simulink model "BatteryTestHarness"  (R2024b)
settings: Solver=VariableStepAuto  StartTime=0.0  StopTime=1200  RelTol=1e-3
libraries: fl_lib x9, nesl_utility x5, simulink x3
settings Model: Creator=jjha  LastModifiedBy=jjha
settings OptimizationCC: ReuseModelBlockBuffer=off
settings RTWCC: GPUComputeCapability=3.5

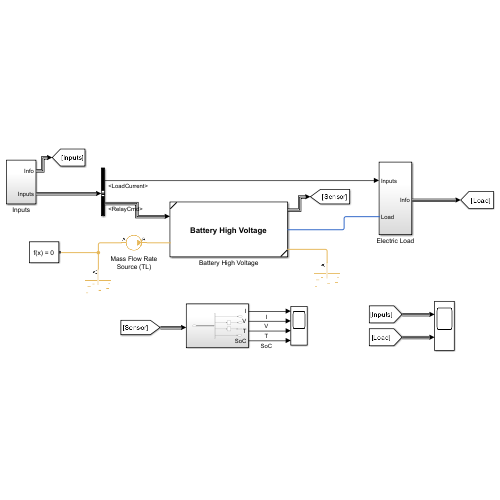
[thumbnail: Simulink's stored preview of the top-level diagram]
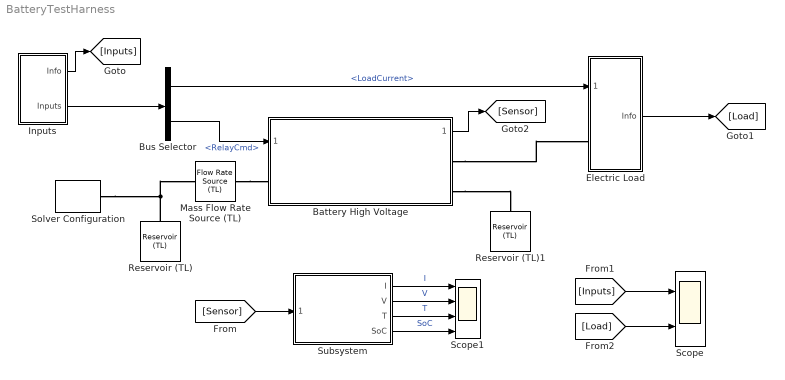
== system BatteryTestHarness ==
  Battery High Voltage : Subsystem  ReferencedSubsystem=BatteryLumpedThermal
      settings: PortSchema="{\"entries\":[{\"content\":{\"sides\":[{\"content\":{\"connectorIds\":[\"In1\",\"LConn1\"]},\"type\":\"ConnectorPlacement.EquallySpacedRectSide\",\"uuid\":\"8181cb02-9fda-4117-b6cc-20d3aa3c91ff\"},{\"content\":{\"connectorIds\":[\"Out1\",\"RConn2\",\"RConn1\"],\"side\":\"RIGHT\"},\"type\":\"ConnectorPlacement.EquallySpacedRectSide\",\"uuid\":\"ce8e42be-3e70-4380-b57d-83f3b727ba87\"},{\"content\":{\"side\":\"TOP\"},\"type\":\"ConnectorPlacement.EquallySpacedRectSide\",\"uuid\":\"6a78c74e-aae9-47cc-a28b-5eba05e58917\"}]},\"type\":\"ConnectorPlacement.EquallySpacedConnector\",\"uuid\":\"1e62e78b-c719-4766-a217-65142f12f1bd\"}],\"packageUris\":[\"http://schema.mathworks.com/mf0/Connector/R2020b\"],\"version\":\"1.0\"}"
  Bus Selector : BusSelector  OutputSignals=Load.LoadCurrent,RelayCmd
  Electric Load : Subsystem
  Inputs : Subsystem
  Mass Flow Rate Source (TL) : fl_lib/Thermal Liquid/Sources/Flow Rate Source (TL)  source_type=foundation.enum.constant_controlled.constant  flow_type=foundation.enum.mass_volumetric_flow.mass  mass_flow=0.001 kg/s  volumetric_flow=0 m^3/s  power_spec=foundation.enum.power_spec.isentropic  area=0.01 m^2
      settings: InternalSimscapePortConfiguration="{\"Bottom\":[],\"Left\":[{\"id\":\"A\",\"label\":\"A\",\"type\":\"foundation.thermal_liquid.thermal_liquid\"}],\"Right\":[{\"id\":\"B\",\"label\":\"B\",\"type\":\"foundation.thermal_liquid.thermal_liquid\"}],\"Top\":[]}"
  Reservoir (TL) : fl_lib/Thermal Liquid/Elements/Reservoir (TL)  pressure_spec=foundation.enum.pressure_spec.atmospheric  reservoir_pressure=0.101325 MPa  reservoir_temperature=293.15 K  area=0.01 m^2
  Reservoir (TL)1 : fl_lib/Thermal Liquid/Elements/Reservoir (TL)  pressure_spec=foundation.enum.pressure_spec.atmospheric  reservoir_pressure=0.101325 MPa  reservoir_temperature=293.15 K  area=0.01 m^2
  Scope : Scope  NumInputPorts=2
  Scope1 : Scope  NumInputPorts=4
  Solver Configuration : nesl_utility/Solver Configuration  PhysicalDomain=network_engine_domain  SubClassName=solver  LeftPortType=input  RightPortType=generic  Tones=[]  Harmonics=[]  SimulateNoise=off  Profile=off  UseLocalSampling=off  EnableSwitchedLinearOptims=on  FrequencyDomain=off  UseCCode=off  RelTol=0.001  AbsTol=0.001  MinStep=1e-09  ToWorkspace=off  RevertToSquareIcSolve=off  NumHomotopyIterations=100  PhasorMode=off  PhasorModeNumHarmonics=1  ConsistencySolver=NEWTON_XTOL_AFTER_FTOL  IndexReductionMethod=DerivativeReplacement  DoDC=off  ResidualTolerance=1e-09  ConsistencyTolSource=GLOBAL  ConsistencyAbsTol=0.001  ConsistencyRelTol=0.001  ConsistencyTolFactor=0.001  UseLocalSolver=off  LocalSolverChoice=NE_BACKWARD_EULER_ADVANCER  ResolveIndetEquations=on  FunctionEvalNumThread=1  LocalSolverSampleTime=0.001  DoFixedCost=off  MaxNonlinIter=3  MaxModeIter=2  ComputeImpulses=off  ImpulseIterations=2  LinearAlgebra=auto  LinearAlgebraNumThread=0  EquationFormulation=NE_TIME_EF  DelaysMemoryBudget=1024  AutomaticFiltering=on  FilteringTimeConstant=0.001  PartitionStorageMethod=AS_NEEDED  PartitionMemoryBudget=1024  PartitionMethod=ROBUST  MultibodyUseLocalSolver=off  MultibodyLocalSolverChoice=ODE1  MultibodyLocalSolverSampleTime=0.001
  Subsystem : Subsystem
  wires:
  Inputs/2(Inputs) -> Bus Selector/1
  Bus Selector/2 -> Battery High Voltage/1  "<RelayCmd>"
  Bus Selector/1 -> Electric Load/1(Inputs)  "<LoadCurrent>"
  Inputs/1(Info) -> [Inputs]
  Electric Load/1(Info) -> [Load]
  Battery High Voltage/1 -> [Sensor]
  [Inputs] -> Scope/1
  [Load] -> Scope/2
  [Sensor] -> Subsystem/1(" ")
  Subsystem/1(I) -> Scope1/1  "I"
  Subsystem/2(V) -> Scope1/2  "V"
  Subsystem/3(T) -> Scope1/3  "T"
  Subsystem/4(SoC) -> Scope1/4  "SoC"
  connections:
  Battery High Voltage/RConn2 -- Electric Load/LConn1
  Mass Flow Rate Source (TL)/RConn1 -- Battery High Voltage/LConn1
  Battery High Voltage/RConn1 -- Reservoir (TL)1/LConn1
  Reservoir (TL)/LConn1 -- Solver Configuration/RConn1 -- Mass Flow Rate Source (TL)/LConn1

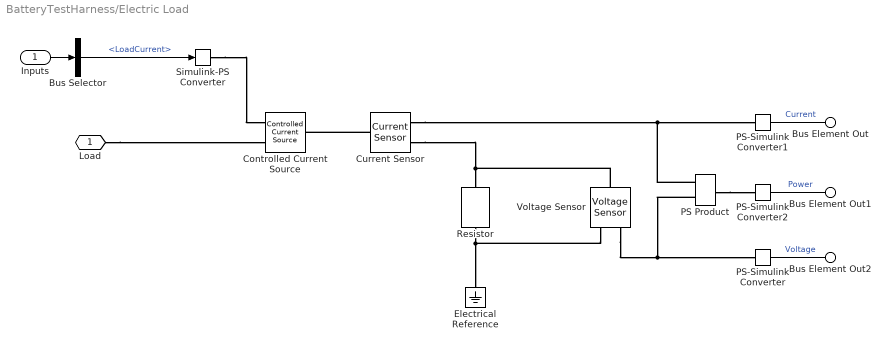
== system BatteryTestHarness/Electric Load ==
  Inputs : Inport
  Bus Selector : BusSelector  OutputSignals=LoadCurrent
  Controlled Current Source : fl_lib/Electrical/Electrical Sources/Controlled Current Source
  Current Sensor : fl_lib/Electrical/Electrical Sensors/Current Sensor
  Electrical Reference : fl_lib/Electrical/Electrical Elements/Electrical Reference
  PS Product : fl_lib/Physical Signals/Functions/PS Product
  PS-Simulink Converter : nesl_utility/PS-Simulink Converter  PhysicalDomain=network_engine_domain  SubClassName=ps_output  LeftPortType=input  RightPortType=output  PseudoPeriodic=off  Frequencies=[]  VectorFormat=inherit  Unit=V  AffineConversion=off
  PS-Simulink Converter1 : nesl_utility/PS-Simulink Converter  PhysicalDomain=network_engine_domain  SubClassName=ps_output  LeftPortType=input  RightPortType=output  PseudoPeriodic=off  Frequencies=[]  VectorFormat=inherit  Unit=A  AffineConversion=off
  PS-Simulink Converter2 : nesl_utility/PS-Simulink Converter  PhysicalDomain=network_engine_domain  SubClassName=ps_output  LeftPortType=input  RightPortType=output  PseudoPeriodic=off  Frequencies=[]  VectorFormat=inherit  Unit=kW  AffineConversion=off
  Resistor : fl_lib/Electrical/Electrical Elements/Resistor  R=1 Ohm  i_specify=off  i_priority=None  i=0 A  i_nominal_specify=off  i_nominal_value=1  i_nominal_unit=A  v_specify=off  v_priority=None  v=0 V  v_nominal_specify=off  v_nominal_value=1  v_nominal_unit=V
  Simulink-PS Converter : nesl_utility/Simulink-PS Converter  PhysicalDomain=network_engine_domain  SubClassName=ps_input  LeftPortType=input  RightPortType=output  PseudoPeriodic=off  Frequencies=[]  NoiseDistribution=none  NoiseParameters=[]  Unit=A  AffineConversion=off  FilteringAndDerivatives=provide  SimscapeFilterOrder=1  InputFilterTimeConstant=0.001  UdotUserProvided=0
  Voltage Sensor : fl_lib/Electrical/Electrical Sensors/Voltage Sensor
  Load : PMIOPort  Side=Left
  Bus Element Out : Outport  PortName=Info  Element=Curr
  Bus Element Out1 : Outport  PortName=Info  Element=Pwr
  Bus Element Out2 : Outport  PortName=Info  Element=V
  wires:
  PS-Simulink Converter1/1 -> Bus Element Out/1  "Current"
  PS-Simulink Converter2/1 -> Bus Element Out1/1  "Power"
  PS-Simulink Converter/1 -> Bus Element Out2/1  "Voltage"
  Inputs/1 -> Bus Selector/1
  Bus Selector/1 -> Simulink-PS Converter/1  "<LoadCurrent>"
  connections:
  Load/RConn1 -- Controlled Current Source/RConn2
  Resistor/RConn1 -- Electrical Reference/LConn1 -- Voltage Sensor/RConn2
  Simulink-PS Converter/RConn1 -- Controlled Current Source/RConn1
  Current Sensor/LConn1 -- Controlled Current Source/LConn1
  Current Sensor/RConn2 -- Voltage Sensor/LConn1 -- Resistor/LConn1
  Voltage Sensor/RConn1 -- PS Product/LConn2 -- PS-Simulink Converter/LConn1
  Current Sensor/RConn1 -- PS Product/LConn1 -- PS-Simulink Converter1/LConn1
  PS Product/RConn1 -- PS-Simulink Converter2/LConn1

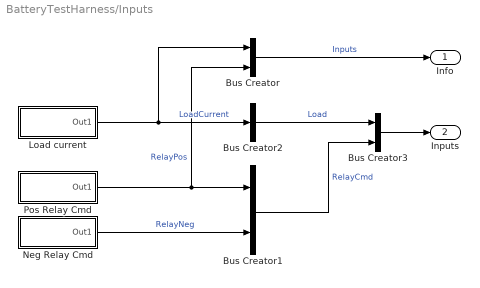
== system BatteryTestHarness/Inputs ==
  Bus Creator : BusCreator  Inputs=2
  Bus Creator1 : BusCreator  Inputs=2
  Bus Creator2 : BusCreator  Inputs=1
  Bus Creator3 : BusCreator  Inputs=2
  Load current : Subsystem  mask(Continuous Multi-Step Signal){dataPoints=[0 5 0;16 114 5;137 256 5;268 378 2;402 479 14;496 579 5;593 660 28;675 787 4;809 901 17;919 1037 25;1049 1137 26;1147 1157 0], deltaT=0.5}
      mask prompts: dataPoints "Data points"; deltaT "Interpolation step [s]"
      mask help:
      | This block generates a signal consisting of smoothly connected flat segments. Data points parameter takes an N-by-3 matrix where each row specifies a flat segment. First column and second column define start and end time of the segment, respectively. Third column defines the value of the segment. Second column can also be NaN to define a point value. Flat segments and point values are smoothly interpolated by Akima spline with the specified interpolation step.
      |
      | For example, a matrix [0 1 5; 3 nan 9; 6 8 7] for Data points defines a signal as follows. First row defines a flat segment from t=0 to t=1 of value 5. Second row defines a point at t=3 of value 9. Third row defines a flat segment from t=6 to t=8 of value 7.
      mask init:
      | sig = SignalDesigner("ContinuousMultiStep");
      | 
      | % Initialization function can access parameter names directly
      | sig.XYData = dataPoints;
      | sig.DeltaX = deltaT;
      | 
      | update(sig)
      | 
      | SignalSourceBlockCallback.setDataToLookupTableBlock( ...
      |   SignalObject = sig, ...
      |   PathToBlock = [gcb '/1-D Lookup Table']);
      mask DialogControl Control3 Prompt: horizontal spacer 1
      mask DialogControl Control4 Prompt: horizontal spacer 2
      mask DialogControl Control5 Prompt: horizontal spacer 3
      mask DialogControl PlotButton Prompt: Plot
      mask DialogControl PlotButton Callback: SignalSourceBlockCallback.plotContinuousMultiStep(gcb);
      mask Display: disp("Continuous" + newline + "Multi-Step")
  Neg Relay Cmd : Subsystem  mask(Continuous Multi-Step Signal){dataPoints=[0 1 0;2 10 1], deltaT=0.1}
      mask prompts: dataPoints "Data points"; deltaT "Interpolation step [s]"
      mask help:
      | This block generates a signal consisting of smoothly connected flat segments. Data points parameter takes an N-by-3 matrix where each row specifies a flat segment. First column and second column define start and end time of the segment, respectively. Third column defines the value of the segment. Second column can also be NaN to define a point value. Flat segments and point values are smoothly interpolated by Akima spline with the specified interpolation step.
      |
      | For example, a matrix [0 1 5; 3 nan 9; 6 8 7] for Data points defines a signal as follows. First row defines a flat segment from t=0 to t=1 of value 5. Second row defines a point at t=3 of value 9. Third row defines a flat segment from t=6 to t=8 of value 7.
      mask init: same as BatteryTestHarness/Inputs/Load current
      mask DialogControl Control3 Prompt: horizontal spacer 1
      mask DialogControl Control4 Prompt: horizontal spacer 2
      mask DialogControl Control5 Prompt: horizontal spacer 3
      mask DialogControl PlotButton Prompt: Plot
      mask DialogControl PlotButton Callback: SignalSourceBlockCallback.plotContinuousMultiStep(gcb);
      mask Display: disp("Continuous" + newline + "Multi-Step")
  Pos Relay Cmd : Subsystem  mask(Continuous Multi-Step Signal){dataPoints=[0 1 0;2 10 1], deltaT=0.1}
      mask prompts: dataPoints "Data points"; deltaT "Interpolation step [s]"
      mask help:
      | This block generates a signal consisting of smoothly connected flat segments. Data points parameter takes an N-by-3 matrix where each row specifies a flat segment. First column and second column define start and end time of the segment, respectively. Third column defines the value of the segment. Second column can also be NaN to define a point value. Flat segments and point values are smoothly interpolated by Akima spline with the specified interpolation step.
      |
      | For example, a matrix [0 1 5; 3 nan 9; 6 8 7] for Data points defines a signal as follows. First row defines a flat segment from t=0 to t=1 of value 5. Second row defines a point at t=3 of value 9. Third row defines a flat segment from t=6 to t=8 of value 7.
      mask init: same as BatteryTestHarness/Inputs/Load current
      mask DialogControl Control3 Prompt: horizontal spacer 1
      mask DialogControl Control4 Prompt: horizontal spacer 2
      mask DialogControl Control5 Prompt: horizontal spacer 3
      mask DialogControl PlotButton Prompt: Plot
      mask DialogControl PlotButton Callback: SignalSourceBlockCallback.plotContinuousMultiStep(gcb);
      mask Display: disp("Continuous" + newline + "Multi-Step")
  Info : Outport
  Inputs : Outport  Port=2
  wires:
  Load current/1(Out1) -> Bus Creator2/1, Bus Creator/1  "LoadCurrent"
  Pos Relay Cmd/1(Out1) -> Bus Creator1/1, Bus Creator/2  "RelayPos"
  Bus Creator/1 -> Info/1  "Inputs"
  Bus Creator2/1 -> Bus Creator3/1  "Load"
  Bus Creator1/1 -> Bus Creator3/2  "RelayCmd"
  Bus Creator3/1 -> Inputs/1
  Neg Relay Cmd/1(Out1) -> Bus Creator1/2  "RelayNeg"

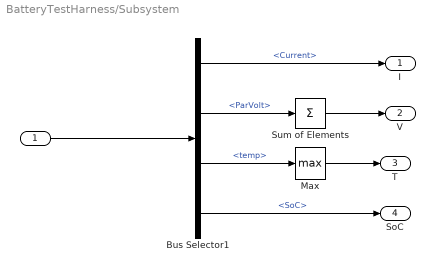
== system BatteryTestHarness/Subsystem ==
  " " : Inport
  Bus Selector1 : BusSelector  OutputSignals=BattSens.Current,BattSens.ParVolt,BattSens.temp,BattSens.SoC
  Max : MinMax  Function=max  ZeroCross=off
  Sum of Elements : Sum  Inputs=+
  I : Outport
  V : Outport  Port=2
  T : Outport  Port=3
  SoC : Outport  Port=4
  wires:
  " "/1 -> Bus Selector1/1
  Bus Selector1/1 -> I/1  "<Current>"
  Bus Selector1/2 -> Sum of Elements/1  "<ParVolt>"
  Bus Selector1/3 -> Max/1  "<temp>"
  Bus Selector1/4 -> SoC/1  "<SoC>"
  Sum of Elements/1 -> V/1
  Max/1 -> T/1

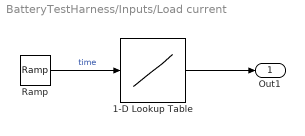
== system BatteryTestHarness/Inputs/Load current ==
  1-D Lookup Table : Lookup_n-D  NumberOfTableDimensions=1  BreakpointsForDimension1="[0              5            5.5              6            6.5              7            7.5              8            8.5              9            9.5             10           10.5             11           11.5             12           12.5             13           13.5             14           14.5             15           15.5             16            114          114.5            115          115.5            116          116.5            117          117.5            118          118.5            119          119.5            120          120.5            121          121.5            122          122.5            123          123.5            124          124.5            125          125.5            126          126.5            127          127.5            128          128.5            129          129.5            130          130.5            131          131.5            132          132.5            133          133.5            134          134.5            135          135.5            136          136.5            137            256          256.5            257          257.5            258          258.5            259          259.5            260          260.5            261          261.5            262          262.5            263          263.5            264          264.5            265          265.5            266          266.5            267          267.5            268            378          378.5            379          379.5            380          380.5            381          381.5            382          382.5            383          383.5            384          384.5            385          385.5            386          386.5            387          387.5            388          388.5            389          389.5            390          390.5            391          391.5            392          392.5            393          393.5            394          394.5            395          395.5            396          396.5            397          397.5            398          398.5            399          399.5            400          400.5            401          401.5            402            479          479.5            480          480.5            481          481.5            482          482.5            483          483.5            484          484.5            485          485.5            486          486.5            487          487.5            488          488.5            489          489.5            490          490.5            491          491.5            492          492.5            493          493.5            494          494.5            495          495.5            496            579          579.5            580          580.5            581          581.5            582          582.5            583          583.5            584          584.5            585          585.5            586          586.5            587          587.5            588          588.5            589          589.5            590          590.5            591          591.5            592          592.5            593            660          660.5            661          661.5            662          662.5            663          663.5            664          664.5            665          665.5            666          666.5            667          667.5            668          668.5            669          669.5            670          670.5            671          671.5            672          672.5            673          673.5            674          674.5            675            787          787.5            788          788.5            789          789.5            790          790.5            791          791.5            792          792.5            793          793.5            794          794.5            795          795.5            796          796.5            797          797.5            798          798.5            799          799.5            800 ...(+1523 chars)]"  Table="[0            0    0.0300526     0.116454     0.253569     0.435763       0.6574     0.912847      1.19647      1.50263      1.82569      2.16003          2.5      2.83997      3.17431      3.49737      3.80353      4.08715       4.3426      4.56424      4.74643      4.88355      4.96995            5            5            5            5            5            5            5            5            5            5            5            5            5            5            5            5            5            5            5            5            5            5            5            5            5            5            5            5            5            5            5            5            5            5            5            5            5            5            5            5            5            5            5            5            5            5            5            5            5      4.98481      4.94097      4.87109      4.77778      4.66363      4.53125      4.38325      4.22222      4.05078      3.87153      3.68707          3.5      3.31293      3.12847      2.94922      2.77778      2.61675      2.46875      2.33637      2.22222      2.12891      2.05903      2.01519            2            2      2.01541      2.06076      2.13477      2.23611       2.3635      2.51562      2.69119      2.88889      3.10742      3.34549      3.60178        3.875      4.16385      4.46701       4.7832      5.11111      5.44944      5.79688      6.15213      6.51389      6.88086      7.25174      7.62522            8      8.37478      8.74826      9.11914      9.48611      9.84787      10.2031      10.5506      10.8889      11.2168       11.533      11.8362       12.125      12.3982      12.6545      12.8926      13.1111      13.3088      13.4844      13.6365      13.7639      13.8652      13.9392      13.9846           14           14      13.9771      13.9102      13.8022      13.6556      13.4733      13.2581      13.0126      12.7397       12.442      12.1223      11.7834       11.428      11.0589      10.6788      10.2905       9.8966          9.5       9.1034      8.70955      8.32119      7.94107      7.57195      7.21657      6.87767      6.55801      6.26033      5.98738      5.74191      5.52666      5.34439      5.19784      5.08976       5.0229            5            5      5.08591      5.33528      5.73551      6.27405      6.93832      7.71574      8.59375      9.55977      10.6012      11.7055      12.8601      14.0525        15.27         16.5        17.73      18.9475      20.1399      21.2945      22.3988      23.4402      24.4062      25.2843      26.0617      26.7259      27.2645      27.6647      27.9141           28           28      27.9218      27.6942       27.328      26.8338      26.2222       25.504      24.6898      23.7902       22.816      21.7778      20.6862       19.552      18.3858      17.1982           16      14.8018      13.6142       12.448      11.3138      10.2222        9.184      8.20978      7.31022        6.496      5.77778      5.16622        4.672      4.30578      4.07822            4            4      4.01984      4.07814      4.17306      4.30278      4.46546      4.65928       4.8824      5.13298      5.40921      5.70924      6.03125       6.3734      6.73387      7.11082      7.50242      7.90684      8.32224      8.74681       9.1787      9.61608      10.0571         10.5      10.9429      11.3839      11.8213      12.2532      12.6778      13.0932      13.4976      13.8892      14.2661      14.6266      14.9688      15.2908      15.5908       15.867      16.1176      16.3407      16.5345      16.6972      16.8269      16.9219      16.9802           17           17      17.0182      17.0713      17.1574      17.2743      17.4201      17.5926      17.7898      18.0096        18.25      18.5089      18.7843      19.0741      19.3762      19.6886      20.0093      20.3361       20.667           21       21.333      21.6639      21.9907      22.3114 ...(+788 chars)]"  InternalRulePriority=Speed  RndMeth=Simplest
  Ramp : simulink/Sources/Ramp  slope=1  start=0  InitialOutput=0
      settings: AttributesFormatString=|
      | Slope: %<slope>
      | Start time: %<start>
      | Initial output: %<InitialOutput>
  Out1 : Outport
  wires:
  Ramp/1 -> 1-D Lookup Table/1  "time"
  1-D Lookup Table/1 -> Out1/1

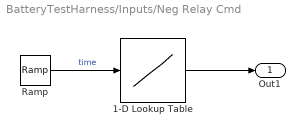
== system BatteryTestHarness/Inputs/Neg Relay Cmd ==
  1-D Lookup Table : Lookup_n-D  NumberOfTableDimensions=1  BreakpointsForDimension1="[0            1          1.1          1.2          1.3          1.4          1.5          1.6          1.7          1.8          1.9            2           10]"  Table="[0           0       0.028       0.104       0.216       0.352         0.5       0.648       0.784       0.896       0.972           1           1]"  InternalRulePriority=Speed  RndMeth=Simplest
  Ramp : simulink/Sources/Ramp  slope=1  start=0  InitialOutput=0
      settings: AttributesFormatString=|
      | Slope: %<slope>
      | Start time: %<start>
      | Initial output: %<InitialOutput>
  Out1 : Outport
  wires:
  1-D Lookup Table/1 -> Out1/1
  Ramp/1 -> 1-D Lookup Table/1  "time"

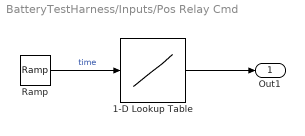
== system BatteryTestHarness/Inputs/Pos Relay Cmd ==
  1-D Lookup Table : Lookup_n-D  NumberOfTableDimensions=1  BreakpointsForDimension1="[0            1          1.1          1.2          1.3          1.4          1.5          1.6          1.7          1.8          1.9            2           10]"  Table="[0           0       0.028       0.104       0.216       0.352         0.5       0.648       0.784       0.896       0.972           1           1]"  InternalRulePriority=Speed  RndMeth=Simplest
  Ramp : simulink/Sources/Ramp  slope=1  start=0  InitialOutput=0
      settings: AttributesFormatString=|
      | Slope: %<slope>
      | Start time: %<start>
      | Initial output: %<InitialOutput>
  Out1 : Outport
  wires:
  Ramp/1 -> 1-D Lookup Table/1  "time"
  1-D Lookup Table/1 -> Out1/1
